simulink model "ex14busSGandPV_sim"  (R2014b)
settings: Solver=ode45  SolverMode=SingleTasking  StartTime=0.0  StopTime=8  MaxStep=0.0008  RelTol=0.0001
values from neighbouring files (symbols this model uses):
  Anf = full(Aksi)    [ex14busSGandPV.m]
  baseV = 1e3*mpcA.bus(1,BASE_KV)    [ex14busSGandPV.m]    (also in ex9busSG_data.mat = 345000; exDroopA.m = 1e3*mpc.bus(:,BASE_KV); exDroopB.m = 1e3*mpc.bus(:,BASE_KV); exLargeSysStability.m = 1e3*mpc.bus(:,BASE_KV))
  Bnf = full(Bksi)    [ex14busSGandPV.m]
  bus1_vd = 2^0.5*1e3    (= 1414.21356237)    [ex3busPV.m]    (also in exLongLinePV.m = 141421.356237)
  Cbus = [600e-6 ; 600e-6]    [ex14busSGandPV.m]    (also in exLongLinePV.m = 0.001)
  Cbus2 = (1e6*mpcC.bus(2,BS))/(ws*baseV^2)    [ex14busSGandPV.m]
  Cbus3 = (1e6*mpcC.bus(3,BS))/(ws*baseV^2)    [ex14busSGandPV.m]
  Cinv = Cinv_pu/(ws*baseZ)    [ex14busSGandPV.m]
  Cnf = full(Cksi)    [ex14busSGandPV.m]
  Dnf = full(Dksi)    [ex14busSGandPV.m]
  If_dc = 0.2*Prt./Ert    [ex14busSGandPV.m]    (also in ex7busLongLine.m = Prt./(60*Vf_dc); exDroopA.m = Prt./(60*Vf_dc); exDroopB.m = Prt./(60*Vf_dc); exSyncGenPVinv.m)
  Kd = KD_GAIN_CNST*J*ws    [ex14busSGandPV.m]    (also in ex2busStability.m = 24000; ex7busLongLine.m; ex9busSG.m; exDroopA.m)
  ki = [0.3 ; 0.3]    [ex14busSGandPV.m]    (also in exLongLinePV.m = 1e-05)
  kp = [1.3e-6 ; 1.3e-6]    [ex14busSGandPV.m]    (also in exLongLinePV.m = 1e-05)
  L0 = 0.1*Ld    [ex14busSGandPV.m]    (also in ex7busLongLine.m; exDroopA.m; exDroopB.m; exSyncGenPVinv.m)
  Laf = (2^0.5)*Ert./(ws*If_dc)    [ex14busSGandPV.m]    (also in ex7busLongLine.m; exDroopA.m; exDroopB.m; exSyncGenPVinv.m = (2^0.5)*5*Ert.^2./(ws*Prt))
  Lb2 = 2*Ld.*Lff - 3*Laf.^2    [ex14busSGandPV.m]    (also in ex7busLongLine.m; exDroopA.m; exDroopB.m; exSyncGenPVinv.m)
  Ld = 0.6*Lpu    [ex14busSGandPV.m]    (also in ex7busLongLine.m = 0.3*Lpu; exDroopA.m = 0.3*Lpu; exDroopB.m = 0.3*Lpu; exSyncGenPVinv.m)
  Lff = 2*Laf.^2./Ld    [ex14busSGandPV.m]    (also in ex7busLongLine.m; exDroopA.m; exDroopB.m; exSyncGenPVinv.m)
  Lq = Ld    [ex14busSGandPV.m]    (also in ex7busLongLine.m; exDroopA.m; exDroopB.m; exSyncGenPVinv.m)
  mpcE = runpf(mpcE)    [ex14busSGandPV.m]    (also in exDroopA.m)
  Nss = length(ssbus)    [ex14busSGandPV.m]
  PG = 2    [ex9busSG_data.mat]
  Pgm = 3*[40; 20]*1e6    [ex14busSGandPV.m]
  poles_2Jws = poles./(2*J*ws)    [ex14busSGandPV.m]    (also in ex2busStability.m = poles./(2*ws*J); ex7busLongLine.m; ex9busSG.m = poles./(2*ws*J); exDroopA.m)
  Pren = [10 ; 10]*1e6    [ex14busSGandPV.m]    (also in ex3busPV.m = 500; exLongLinePV.m = 5000000)
  PT = 16    [ex9busSG_data.mat]
  QG = 3    [ex9busSG_data.mat]
  QT = 17    [ex9busSG_data.mat]
  Ra = 0.05*Ert.^2./Prt    [ex14busSGandPV.m]    (also in ex7busLongLine.m = 0.01*Ert.^2./Prt; exDroopA.m = 0.01*Ert.^2./Prt; exDroopB.m = 0.01*Ert.^2./Prt; exSyncGenPVinv.m)
  Rf = Lff/1.2    [ex14busSGandPV.m]    (also in ex7busLongLine.m = Vf_dc./If_dc; exDroopA.m = Vf_dc./If_dc; exDroopB.m = Vf_dc./If_dc; exSyncGenPVinv.m)
  step_size_bus2 = 0    [ex14busSGandPV.m]
  step_size_bus3 = 0    [ex14busSGandPV.m]
  step_size_bus6 = 0    [ex14busSGandPV.m]
  step_size_bus8 = 0    [ex14busSGandPV.m]
  step_time_bus2 = 3    [ex14busSGandPV.m]
  step_time_bus3 = 3    [ex14busSGandPV.m]
  step_time_bus6 = 5    [ex14busSGandPV.m]
  step_time_bus8 = 5    [ex14busSGandPV.m]
  VA = 9    [ex9busSG_data.mat]
  Vbus_ref = [800 ; 800]    [ex14busSGandPV.m]    (also in exLongLinePV.m = 800)
  Vf_dc = If_dc.*Rf    [ex14busSGandPV.m]    (also in ex7busLongLine.m = 500 * ones(size(Ert)); exDroopA.m = 500 * ones(size(Ert)); exDroopB.m = 500 * ones(size(Ert)); exSyncGenPVinv.m)
  vinf_0 = 0    [ex14busSGandPV.m]    (also in ex7busLongLine.m; exDroopA.m; exSyncGenPVinv.m)
  vinf_d = (2^0.5)*mpcA.bus(1,VM)*baseV    [ex14busSGandPV.m]    (also in ex7busLongLine.m = 250457.221896; exDroopA.m = (2^0.5)*mpc.bus(1,VM)*baseV(1); exSyncGenPVinv.m = (2^0.5)*mpc.bus(1,VM)*baseV(1))
  vinf_q = 0    [ex14busSGandPV.m]    (also in ex7busLongLine.m; exDroopA.m; exSyncGenPVinv.m)
  vinit_dq0_bus2 = [real(vpp) ; imag(vpp) ; 0]    [ex14busSGandPV.m]
  vinit_dq0_bus3 = [real(vpp) ; imag(vpp) ; 0]    [ex14busSGandPV.m]
  vinit_dq0_bus6 = [real(vpp) ; imag(vpp) ; 0]    [ex14busSGandPV.m]
  vinit_dq0_bus8 = [real(vpp) ; imag(vpp) ; 0]    [ex14busSGandPV.m]
  VM = 8    [ex9busSG_data.mat]
  ws = 2*pi*50    (= 314.159265359)    [ex14busSGandPV.m]    (also in ex2busStability.m; ex3busPV.m; ex7busLongLine.m; ex9busSG.m)
libraries: simulink x2
(part 2 of 2)

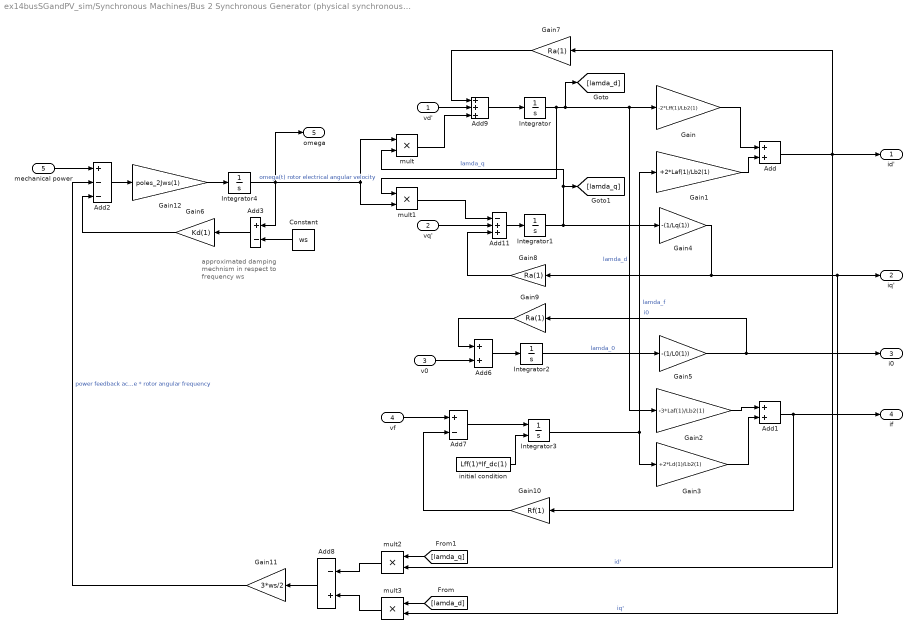
== system ex14busSGandPV_sim/Synchronous Machines/Bus 2 Synchronous Generator (physical synchronous machine model)/synchronous machine dq0 model reference angle is teta(t) = rotor electrical angle ==
  note: approximated damping
      | mechnism in respect to
      | frequency ws
  vd' : Inport
  vq' : Inport  Port=2
  v0 : Inport  Port=3
  vf : Inport  Port=4
  mechanical power : Inport  Port=5
  Add : Sum
  Add1 : Sum
  Add11 : Sum  Inputs=-++
  Add2 : Sum  Inputs=+--
  Add3 : Sum  Inputs=+-
  Add6 : Sum
  Add7 : Sum  Inputs=+-
  Add8 : Sum  Inputs=-+
  Add9 : Sum  Inputs=+++
  Constant : Constant  Value=ws
  Gain : Gain  Gain=-2*Lff(1)/Lb2(1)
  Gain1 : Gain  Gain=+2*Laf(1)/Lb2(1)
  Gain10 : Gain  Gain=Rf(1)
  Gain11 : Gain  Gain=3*ws/2
  Gain12 : Gain  Gain=poles_2Jws(1)
  Gain2 : Gain  Gain=-3*Laf(1)/Lb2(1)
  Gain3 : Gain  Gain=+2*Ld(1)/Lb2(1)
  Gain4 : Gain  Gain=-(1/Lq(1))
  Gain5 : Gain  Gain=-(1/L0(1))
  Gain6 : Gain  Gain=Kd(1)
  Gain7 : Gain  Gain=Ra(1)
  Gain8 : Gain  Gain=Ra(1)
  Gain9 : Gain  Gain=Ra(1)
  Integrator : Integrator
  Integrator1 : Integrator
  Integrator2 : Integrator
  Integrator3 : Integrator  InitialConditionSource=external  InitialCondition=Lff(1)*If_dc(1)
  Integrator4 : Integrator  InitialCondition=ws
  initial condition : Constant  Value=Lff(1)*If_dc(1)
  mult{,1..3} (4 alike) : Product  Inputs=**
  id' : Outport
  iq' : Outport  Port=2
  i0 : Outport  Port=3
  if : Outport  Port=4
  omega : Outport  Port=5
  wires:
  Gain1/1 -> Add/2
  Add6/1 -> Integrator2/1
  mechanical power/1 -> Add2/1
  Gain6/1 -> Add2/3
  Integrator/1 -> mult1/1, Gain2/1, Gain/1, [lamda_d]  "lamda_d"
  Gain5/1 -> i0/1, Gain9/1  "i0"
  Integrator1/1 -> Gain4/1, [lamda_q], mult/2  "lamda_q"
  Integrator2/1 -> Gain5/1  "lamda_0"
  Integrator3/1 -> Gain1/1, Gain3/1  "lamda_f"
  Add1/1 -> if/1, Gain10/1
  Gain4/1 -> iq'/1, mult3/2, Gain8/1  "iq'"
  Add/1 -> mult2/2, id'/1, Gain7/1  "id'"
  Gain/1 -> Add/1
  vf/1 -> Add7/1
  Add7/1 -> Integrator3/1
  Gain9/1 -> Add6/1
  Add8/1 -> Gain11/1
  Gain11/1 -> Add2/2  "power feedback acting to slow the rotor = Torque * rotor angular frequency"
  Gain8/1 -> Add11/3
  mult/1 -> Add9/3
  mult1/1 -> Add11/1
  Add9/1 -> Integrator/1
  vd'/1 -> Add9/2
  Gain3/1 -> Add1/2
  Gain2/1 -> Add1/1
  Gain10/1 -> Add7/2
  Add11/1 -> Integrator1/1
  Gain7/1 -> Add9/1
  mult3/1 -> Add8/2
  mult2/1 -> Add8/1
  v0/1 -> Add6/2
  Add3/1 -> Gain6/1
  Constant/1 -> Add3/2
  vq'/1 -> Add11/2
  [lamda_q] -> mult2/1
  [lamda_d] -> mult3/1
  Integrator4/1 -> omega/1, Add3/1, mult1/2, mult/1  "omega(t) rotor electrical angular velocity"
  Add2/1 -> Gain12/1
  Gain12/1 -> Integrator4/1
  initial condition/1 -> Integrator3/2

== system ex14busSGandPV_sim/Synchronous Machines/Bus 3 Synchronous Generator (physical synchronous machine model)/measurements ==
  vdq0 : Inport
  idq0 : Inport  Port=2
  Add : Sum  Inputs=+++
  Add1 : Sum  Inputs=+-
  Add2 : Sum
  Demux : Demux  Outputs=3
  Demux1 : Demux  Outputs=3
  Gain : Gain  Gain=0.5
  Gain1 : Gain  Gain=0.5
  Gain2 : Gain  Gain=0.5
  Gain3 : Gain  Gain=2
  Gain4 : Gain  Gain=180/pi
  Math Function : Math  Operator=square  SaturateOnIntegerOverflow=on
  Math Function1 : Math  Operator=square  SaturateOnIntegerOverflow=on
  Sqrt : Sqrt  SaturateOnIntegerOverflow=on
  Trigonometric Function : Trigonometry  Operator=atan2
  mult{,1..4} (5 alike) : Product  Inputs=**
  P : Outport
  Q : Outport  Port=2
  Vm_RMS : Outport  Port=3
  Vph_deg : Outport  Port=4
  wires:
  idq0/1 -> Demux1/1
  vdq0/1 -> Demux/1
  Demux/1 -> Math Function/1, Trigonometric Function/2, mult3/1, mult/1  "vd"
  Demux/2 -> Trigonometric Function/1, Math Function1/1, mult2/1, mult1/1  "vq"
  Demux1/1 -> mult/2, mult2/2  "id"
  Demux1/2 -> mult3/2, mult1/2  "iq"
  Demux/3 -> mult4/1  "v0"
  Demux1/3 -> mult4/2  "i0"
  mult/1 -> Add/1
  mult1/1 -> Add/2
  Add/1 -> Gain/1
  mult2/1 -> Add1/1
  mult3/1 -> Add1/2
  Add1/1 -> Gain1/1
  Sqrt/1 -> Vm_RMS/1
  Math Function/1 -> Add2/1
  Math Function1/1 -> Add2/2
  Add2/1 -> Gain2/1
  Gain2/1 -> Sqrt/1
  Gain/1 -> P/1
  Gain1/1 -> Q/1
  mult4/1 -> Gain3/1
  Gain3/1 -> Add/3
  Trigonometric Function/1 -> Gain4/1
  Gain4/1 -> Vph_deg/1

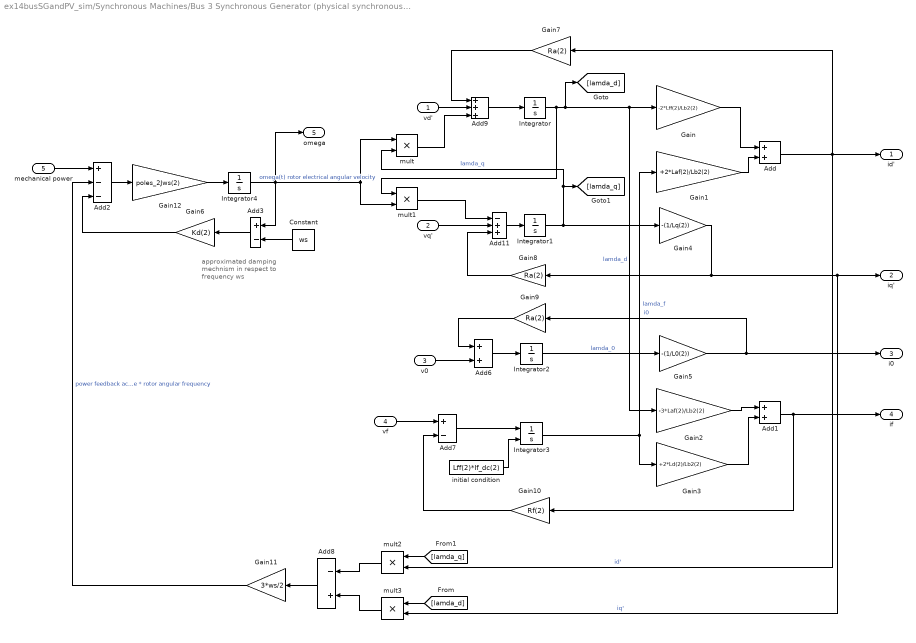
== system ex14busSGandPV_sim/Synchronous Machines/Bus 3 Synchronous Generator (physical synchronous machine model)/synchronous machine dq0 model reference angle is teta(t) = rotor electrical angle ==
  note: approximated damping
      | mechnism in respect to
      | frequency ws
  vd' : Inport
  vq' : Inport  Port=2
  v0 : Inport  Port=3
  vf : Inport  Port=4
  mechanical power : Inport  Port=5
  Add : Sum
  Add1 : Sum
  Add11 : Sum  Inputs=-++
  Add2 : Sum  Inputs=+--
  Add3 : Sum  Inputs=+-
  Add6 : Sum
  Add7 : Sum  Inputs=+-
  Add8 : Sum  Inputs=-+
  Add9 : Sum  Inputs=+++
  Constant : Constant  Value=ws
  Gain : Gain  Gain=-2*Lff(2)/Lb2(2)
  Gain1 : Gain  Gain=+2*Laf(2)/Lb2(2)
  Gain10 : Gain  Gain=Rf(2)
  Gain11 : Gain  Gain=3*ws/2
  Gain12 : Gain  Gain=poles_2Jws(2)
  Gain2 : Gain  Gain=-3*Laf(2)/Lb2(2)
  Gain3 : Gain  Gain=+2*Ld(2)/Lb2(2)
  Gain4 : Gain  Gain=-(1/Lq(2))
  Gain5 : Gain  Gain=-(1/L0(2))
  Gain6 : Gain  Gain=Kd(2)
  Gain7 : Gain  Gain=Ra(2)
  Gain8 : Gain  Gain=Ra(2)
  Gain9 : Gain  Gain=Ra(2)
  Integrator : Integrator
  Integrator1 : Integrator
  Integrator2 : Integrator
  Integrator3 : Integrator  InitialConditionSource=external  InitialCondition=Lff(1)*If_dc(1)
  Integrator4 : Integrator  InitialCondition=ws
  initial condition : Constant  Value=Lff(2)*If_dc(2)
  mult{,1..3} (4 alike) : Product  Inputs=**
  id' : Outport
  iq' : Outport  Port=2
  i0 : Outport  Port=3
  if : Outport  Port=4
  omega : Outport  Port=5
  wires:
  Gain1/1 -> Add/2
  Add6/1 -> Integrator2/1
  mechanical power/1 -> Add2/1
  Gain6/1 -> Add2/3
  Integrator/1 -> mult1/1, Gain2/1, Gain/1, [lamda_d]  "lamda_d"
  Gain5/1 -> i0/1, Gain9/1  "i0"
  Integrator1/1 -> Gain4/1, [lamda_q], mult/2  "lamda_q"
  Integrator2/1 -> Gain5/1  "lamda_0"
  Integrator3/1 -> Gain3/1, Gain1/1  "lamda_f"
  Add1/1 -> if/1, Gain10/1
  Gain4/1 -> iq'/1, mult3/2, Gain8/1  "iq'"
  Add/1 -> mult2/2, id'/1, Gain7/1  "id'"
  Gain/1 -> Add/1
  vf/1 -> Add7/1
  Add7/1 -> Integrator3/1
  Gain9/1 -> Add6/1
  Add8/1 -> Gain11/1
  Gain11/1 -> Add2/2  "power feedback acting to slow the rotor = Torque * rotor angular frequency"
  Gain8/1 -> Add11/3
  mult/1 -> Add9/3
  mult1/1 -> Add11/1
  Add9/1 -> Integrator/1
  vd'/1 -> Add9/2
  Gain3/1 -> Add1/2
  Gain2/1 -> Add1/1
  Gain10/1 -> Add7/2
  Add11/1 -> Integrator1/1
  Gain7/1 -> Add9/1
  mult3/1 -> Add8/2
  mult2/1 -> Add8/1
  v0/1 -> Add6/2
  Add3/1 -> Gain6/1
  Constant/1 -> Add3/2
  vq'/1 -> Add11/2
  [lamda_q] -> mult2/1
  [lamda_d] -> mult3/1
  Integrator4/1 -> omega/1, Add3/1, mult1/2, mult/1  "omega(t) rotor electrical angular velocity"
  Add2/1 -> Gain12/1
  Gain12/1 -> Integrator4/1
  initial condition/1 -> Integrator3/2
